simulink library "THB_set_T"  (Simulink 8.2)
settings: Solver=ode45  StartTime=0.0  StopTime=10.0  RelTol=1e-3
settings Model: Creator=lena.frank  LastModifiedBy=awohlfei

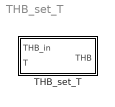
== system THB_set_T ==
  THB_set_T : Subsystem  InitFcn=load('THB.mat');  mask(set temperature in THB){}
      mask help: Set a variable temperature in the thermo-hydraulic bus.
      mask Help: web(['file:///' fullfile(path_carnot('help'),'THB_set_T.html')],'-helpbrowser')

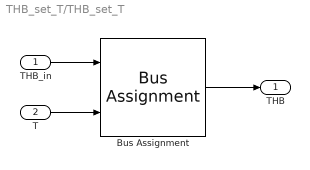
== system THB_set_T/THB_set_T ==
  THB_in : Inport
  T : Inport  Port=2
  Bus Assignment : BusAssignment  AssignedSignals=Temperature
  THB : Outport
  wires:
  T/1 -> Bus Assignment/2
  Bus Assignment/1 -> THB/1
  THB_in/1 -> Bus Assignment/1
